simulink model "doc_design_iteration_viterbi_rayleigh_OFDM_MIMO"  (R2014a)
settings: Solver=FixedStepDiscrete  SolverMode=SingleTasking  StartTime=0.0  StopTime=inf  RelTol=1e-3
PostLoadFcn:
  | if ~exist('EbNo'),EbNo=6;end
  | if ~exist('maxNumBits'),maxNumBits=1e7;end;
  | if ~exist('maxNumErrs'),maxNumErrs=1e3;end;
  | 
  | load Parameters.mat
values from neighbouring files (symbols this model uses):
  EbNo = getTestParameter(obj,'EbNo')    [GrayCodedMod_EbNo_M.m]    (also in GrayCodedModulation2.m; commdoc_code.m = 10; commdoc_gray.m = 10; commdoc_mcurves.m = EbNoVec(idxEbNo))
  Peven = [1.41421356237 0 -1.41421356237 0 1.41421356237 0 -1.41421356237 0 1.41421356237 0 1.41421356237 0 ... (201 elements, 201x1)]    [Parameters.mat]
  Podd = [0 1.41421356237 0 1.41421356237 0 1.41421356237 0 1.41421356237 0 1.41421356237 0 -1.41421356237 ... (201 elements, 201x1)]    [Parameters.mat]
undefined symbols (not defined in the file or in its folder): doppler, prm80216ds
libraries: dspmtrx3 x4, dspindex x3, commchan3 x2, commdigbbndpm3 x2, commofdm x2, commcnvcod2 x2, commmimo x2, dspsigops x2, dspstat3 x1, dspmathops x1, commsink2 x1, commrandsrc2 x1
settings Model: Creator=The MathWorks Inc.
settings OptimizationCC: ExpressionDepthLimit=2147483647
settings DebuggingCC: UnderspecifiedInitializationDetection=Classic  SolverPrmCheckMsg=none  StateNameClashWarn=warning

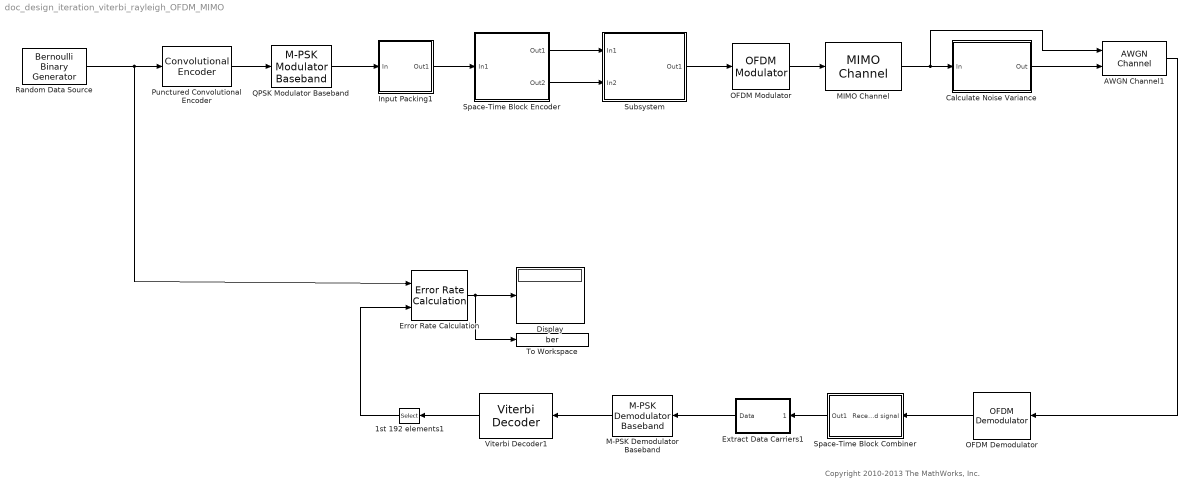
== system doc_design_iteration_viterbi_rayleigh_OFDM_MIMO ==
  note: Copyright 2010-2013 The MathWorks, Inc.
  1st 192 elements1 : Selector  NumberOfDimensions=2  InputPortWidth=3  IndexOptions=Index vector (dialog),Index vector (dialog)  Indices=1:378,1  OutputSizes=1,1
  AWGN Channel1 : commchan3/AWGN Channel  InputProcessing=Columns as channels (frame based)  seed=67  noiseMode=Variance from port  EbNodB=10  EsNodB=15  SNRdB=10  bitsPerSym=1  Ps=1  Tsym=1e-6  variance=1
  Calculate Noise Variance : Subsystem
      mask Display: disp('Calculate\nNoise Variance')
  Display : Display
  Error Rate Calculation : commsink2/Error Rate Calculation  N=0  st_delay=0  cp_mode=Entire frame  subframe=[]  PMode=Port  WsName=ErrorVec1  RsMode2=off  stop=on  numErr=maxNumErrs  maxBits=maxNumBits
  Extract Data Carriers1 : Subsystem  mask(OFDM Receiver){}
      mask Display: disp('Extract\nData Carriers');
  Input Packing1 : Subsystem
      mask Display: disp('IFFT Input\nPacking');
  M-PSK Demodulator Baseband : commdigbbndpm3/M-PSK Demodulator Baseband  M=4  Ph=pi/4  Dec=Gray  Mapping=[0 2 3 1]  OutType=Bit  DecType=Hard decision  VarSource=Dialog  Variance=1  outDtype1=boolean  outDtype2=Inherit via internal rule  derotateFactorWordLen=16
  MIMO Channel : commchan3/MIMO Channel  SimulateUsing=Code generation  SampleRate=3e6/25  PathDelays=[0 0.4 0.9]*1e-6  AveragePathGains=[0 -5 -10]  NormalizePathGains=on  FadingDistribution=Rayleigh  KFactor=3  DirectPathDopplerShift=0  DirectPathInitialPhase=0  MaximumDopplerShift=5  DopplerSpectrum=doppler( 'Jakes' )  SpatialCorrelation=on  NumTransmitAntennas=2  NumReceiveAntennas=1  TransmitCorrelationMatrix=[1 0; 0 1]  ReceiveCorrelationMatrix=1  AntennaSelection=Off  NormalizeChannelOutputs=on  RandomStream=mt19937ar with seed  Seed=73  PathGainsOutputPort=off
  OFDM Demodulator : commofdm/OFDM Demodulator  SimulateUsing=Code generation  FFTLength=256  NumGuardBandCarriers=[28; 27]  RemoveDCCarrier=off  PilotOutputPort=off  PilotCarrierIndices=[12; 26; 40; 54]  CyclicPrefixLength=32  NumSymbols=3  NumReceiveAntennas=1
  OFDM Modulator : commofdm/OFDM Modulator  SimulateUsing=Code generation  FFTLength=256  NumGuardBandCarriers=[28; 27]  InsertDCNull=off  PilotInputPort=off  PilotCarrierIndices=[12; 26; 40; 54]  CyclicPrefixLength=32  Windowing=off  WindowLength=1  NumSymbols=3  NumTransmitAntennas=2
  Punctured Convolutional Encoder : commcnvcod2/Convolutional Encoder  trellis=poly2trellis(7, [171 133])  opMode=Terminate trellis by appending bits  DelayedResetAction=off  hasIniStPort=off  hasFinStPort=off  usePuncVector=on  punctureVector=reshape([1 0;1 1],4,1)  reset=Unused parameter value
  QPSK Modulator Baseband : commdigbbndpm3/M-PSK Modulator Baseband  M=4  InType=Bit  Enc=Gray  Mapping=[0 2 3 1]  Ph=pi/4  outDtype=double  outWordLen=16  outUDDataType=sfix(16)  outFracLenMode=Best precision  outFracLen=15
  Random Data Source : commrandsrc2/Bernoulli Binary Generator  P=0.5  seed=61  Ts=25/3e6  frameBased=on  sampPerFrame=378  orient=off  outDataType=boolean
  Space-Time Block Encoder : Subsystem
      mask Display: disp('Space-Time\nDiversity\nEncoder');
  Space-Time Block Combiner : Subsystem
      mask Display: disp('Space-Time\nDiversity\nCombiner');
  Subsystem : Subsystem
      mask Display: disp('Add OFDM\nPreamble');
  To Workspace : ToWorkspace  VariableName=ber  SampleTime=-1
      settings: MaxDataPoints=1
  Viterbi Decoder1 : commcnvcod2/Viterbi Decoder  trellis=poly2trellis(7, [171 133])  isPunctured=off  punctureVector=reshape([1 0;1 1],4,1)  erasures=off  dectype=Hard decision  runSigValErrCheck=off  nsdecb=4  smWordLength=16  tbdepth=34  opmode=Terminated  reset=off  outDataType=boolean  delayedResetAction=off
  wires:
  Random Data Source/1 -> Error Rate Calculation/1, Punctured Convolutional Encoder/1
  Punctured Convolutional Encoder/1 -> QPSK Modulator Baseband/1
  QPSK Modulator Baseband/1 -> Input Packing1/1(In)
  Extract Data Carriers1/1(Data) -> M-PSK Demodulator Baseband/1
  M-PSK Demodulator Baseband/1 -> Viterbi Decoder1/1
  Viterbi Decoder1/1 -> 1st 192 elements1/1
  Input Packing1/1(Out1) -> Space-Time Block Encoder/1(In1)
  Space-Time Block Combiner/1(Out1) -> Extract Data Carriers1/1(Received signal)
  Error Rate Calculation/1 -> Display/1, To Workspace/1
  1st 192 elements1/1 -> Error Rate Calculation/2
  OFDM Modulator/1 -> MIMO Channel/1
  Subsystem/1(Out1) -> OFDM Modulator/1
  Space-Time Block Encoder/1(Out1) -> Subsystem/1(In1)
  Space-Time Block Encoder/2(Out2) -> Subsystem/2(In2)
  OFDM Demodulator/1 -> Space-Time Block Combiner/1(Received signal)
  MIMO Channel/1 -> Calculate Noise Variance/1(In), AWGN Channel1/1
  Calculate Noise Variance/1(Out) -> AWGN Channel1/2
  AWGN Channel1/1 -> OFDM Demodulator/1

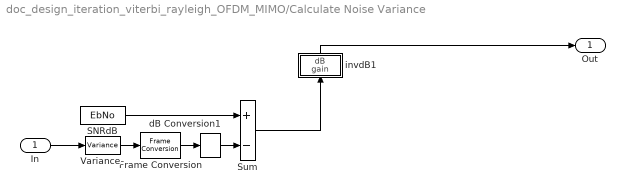
== system doc_design_iteration_viterbi_rayleigh_OFDM_MIMO/Calculate Noise Variance ==
  In : Inport
  Frame Conversion : FrameConversion  OutFrame=Sample-based
  SNRdB : Constant  Value=EbNo
  Sum : Sum  Inputs=+-  SaturateOnIntegerOverflow=on
  Variance : dspstat3/Variance  run=off  reset_popup=None  InputProcessing=Columns as channels (frame based)  directionMode=Each column  dimension=1  treatSBRowAsCol=on  roiEnable=off  roiType=Rectangles  roiPortion=Entire ROI  roiOutput=Individual statistics for each ROI  roiFlag=off  roundingMode=Floor  overflowMode=off
  dB Conversion1 : dspmathops/dB Conversion  dBtype=dB  intype=Power  R=1  fuzz=on
  invdB1 : Subsystem
      mask Display: disp('1/invdB')
  Out : Outport
  wires:
  dB Conversion1/1 -> Sum/2
  Variance/1 -> Frame Conversion/1
  Frame Conversion/1 -> dB Conversion1/1
  invdB1/1(dB) -> Out/1
  Sum/1 -> invdB1/1(gain)
  SNRdB/1 -> Sum/1
  In/1 -> Variance/1

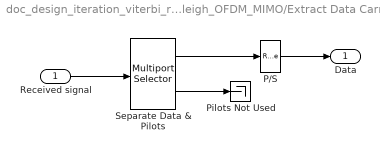
== system doc_design_iteration_viterbi_rayleigh_OFDM_MIMO/Extract Data Carriers1 ==
  Received signal : Inport
  P/S : Reshape  OutputDimensionality=Column vector (2-D)  OutputDimensions=[72, 1]
  Pilots Not Used : Terminator
  Separate Data & Pilots : dspindex/Multiport Selector  rowsOrCols=Rows  idxCellArray={[1:12 14:37 39:62 64:87 89:112 114:137 139:162 164:187 189:200],[13 38 63 88 113 138 163 188]}  idxErrMode=Clip Index
  Data : Outport
  wires:
  Received signal/1 -> Separate Data & Pilots/1
  Separate Data & Pilots/2 -> Pilots Not Used/1
  Separate Data & Pilots/1 -> P/S/1
  P/S/1 -> Data/1

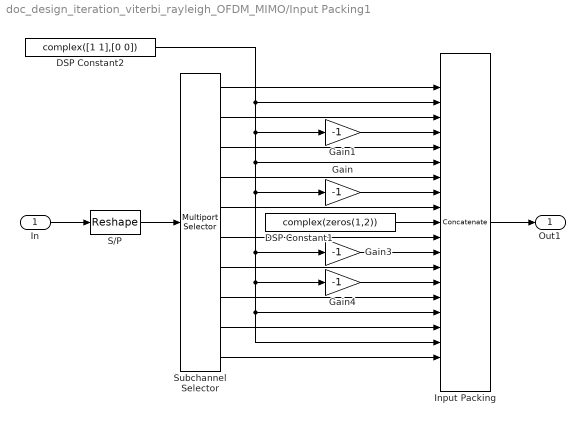
== system doc_design_iteration_viterbi_rayleigh_OFDM_MIMO/Input Packing1 ==
  In : Inport
  DSP Constant1 : Constant  Value=complex(zeros(1,2))  VectorParams1D=off
      settings: SamplingMode=Frame based
  DSP Constant2 : Constant  Value=complex([1 1],[0 0])  VectorParams1D=off
      settings: SamplingMode=Frame based
  Gain{,1,3..4} (4 alike) : Gain  Gain=-1
  Input Packing : Concatenate  NumInputs=19  Mode=Multidimensional array
  S/P : Reshape  OutputDimensionality=Customize  OutputDimensions=[192 2]
  Subchannel Selector : dspindex/Multiport Selector  rowsOrCols=Rows  idxCellArray={[1:12],[13:36],[37:60],[61:84],[85:96],[97:108],[109:132],[133:156],[157:180],[181:192]}  idxErrMode=Generate Error
  Out1 : Outport
  wires:
  Input Packing/1 -> Out1/1
  Gain4/1 -> Input Packing/14
  Gain3/1 -> Input Packing/12
  S/P/1 -> Subchannel Selector/1
  Gain1/1 -> Input Packing/4
  Gain/1 -> Input Packing/8
  DSP Constant1/1 -> Input Packing/10
  Subchannel Selector/1 -> Input Packing/1
  Subchannel Selector/2 -> Input Packing/3
  Subchannel Selector/3 -> Input Packing/5
  Subchannel Selector/4 -> Input Packing/7
  Subchannel Selector/5 -> Input Packing/9
  Subchannel Selector/6 -> Input Packing/11
  Subchannel Selector/7 -> Input Packing/13
  Subchannel Selector/8 -> Input Packing/15
  Subchannel Selector/9 -> Input Packing/17
  Subchannel Selector/10 -> Input Packing/19
  DSP Constant2/1 -> Input Packing/2, Input Packing/6, Gain3/1, Gain4/1, Input Packing/18, Input Packing/16, Gain/1, Gain1/1
  In/1 -> S/P/1

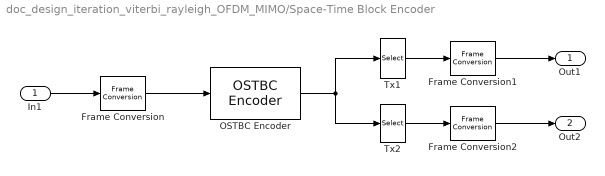
== system doc_design_iteration_viterbi_rayleigh_OFDM_MIMO/Space-Time Block Encoder ==
  In1 : Inport
  Frame Conversion : FrameConversion  OutFrame=Sample-based
  Frame Conversion1 : FrameConversion
  Frame Conversion2 : FrameConversion
  OSTBC Encoder : commmimo/OSTBC Encoder  numTx=2  rate=3/4  overflowMode=Wrap
  Tx1 : Selector  NumberOfDimensions=3  InputPortWidth=256  IndexOptions=Select all,Select all,Index vector (dialog)  Indices=prm80216ds.txCPIndices,1,1  OutputSizes=1,1,1
  Tx2 : Selector  NumberOfDimensions=3  InputPortWidth=256  IndexOptions=Select all,Select all,Index vector (dialog)  Indices=prm80216ds.txCPIndices,1,2  OutputSizes=1,1,1
  Out1 : Outport
  Out2 : Outport  Port=2
  wires:
  In1/1 -> Frame Conversion/1
  Frame Conversion1/1 -> Out1/1
  Frame Conversion2/1 -> Out2/1
  Tx1/1 -> Frame Conversion1/1
  Tx2/1 -> Frame Conversion2/1
  OSTBC Encoder/1 -> Tx1/1, Tx2/1
  Frame Conversion/1 -> OSTBC Encoder/1

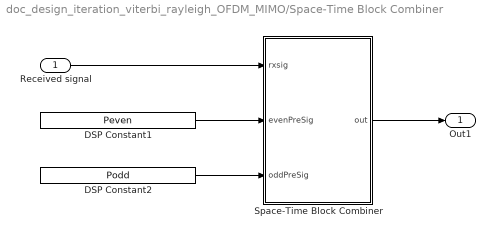
== system doc_design_iteration_viterbi_rayleigh_OFDM_MIMO/Space-Time Block Combiner ==
  Received signal : Inport
  DSP Constant1 : Constant  Value=Peven  VectorParams1D=off
      settings: SamplingMode=Frame based
  DSP Constant2 : Constant  Value=Podd  VectorParams1D=off
      settings: SamplingMode=Frame based
  Space-Time Block Combiner : Subsystem
      mask init:
      | a = [1:100; 1:100];
      mask Display: disp('Channel Estimation\n& Space-Time\nBlock Combining')
  Out1 : Outport
  wires:
  Space-Time Block Combiner/1(out) -> Out1/1
  Received signal/1 -> Space-Time Block Combiner/1(rxsig)
  DSP Constant2/1 -> Space-Time Block Combiner/3(oddPreSig)
  DSP Constant1/1 -> Space-Time Block Combiner/2(evenPreSig)

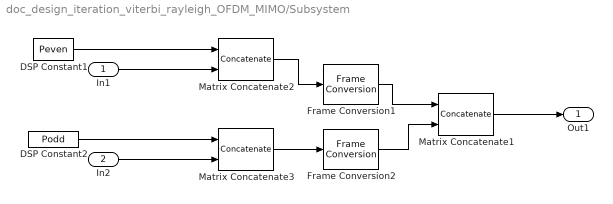
== system doc_design_iteration_viterbi_rayleigh_OFDM_MIMO/Subsystem ==
  In1 : Inport
  In2 : Inport  Port=2
  DSP Constant1 : Constant  Value=Peven  VectorParams1D=off
      settings: SamplingMode=Frame based
  DSP Constant2 : Constant  Value=Podd  VectorParams1D=off
      settings: SamplingMode=Frame based
  Frame Conversion1 : FrameConversion  OutFrame=Sample-based
  Frame Conversion2 : FrameConversion  OutFrame=Sample-based
  Matrix Concatenate1 : Concatenate  Mode=Multidimensional array  ConcatenateDimension=3
  Matrix Concatenate2 : Concatenate  Mode=Multidimensional array  ConcatenateDimension=2
  Matrix Concatenate3 : Concatenate  Mode=Multidimensional array  ConcatenateDimension=2
  Out1 : Outport
  wires:
  In2/1 -> Matrix Concatenate3/2
  In1/1 -> Matrix Concatenate2/2
  Matrix Concatenate1/1 -> Out1/1
  Frame Conversion1/1 -> Matrix Concatenate1/1
  Frame Conversion2/1 -> Matrix Concatenate1/2
  Matrix Concatenate3/1 -> Frame Conversion2/1
  Matrix Concatenate2/1 -> Frame Conversion1/1
  DSP Constant2/1 -> Matrix Concatenate3/1
  DSP Constant1/1 -> Matrix Concatenate2/1

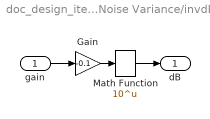
== system doc_design_iteration_viterbi_rayleigh_OFDM_MIMO/Calculate Noise Variance/invdB1 ==
  gain : Inport
  Gain : Gain  Gain=-0.1  SaturateOnIntegerOverflow=on  OutDataTypeStr=Inherit: Same as input  ParamDataTypeStr=Inherit: Same as input
  Math Function : Math  Operator=10^u  SaturateOnIntegerOverflow=on
  dB : Outport
  wires:
  Gain/1 -> Math Function/1
  gain/1 -> Gain/1
  Math Function/1 -> dB/1

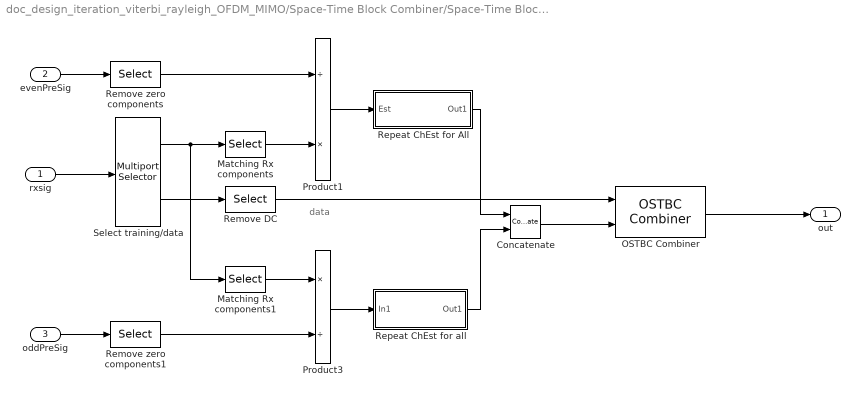
== system doc_design_iteration_viterbi_rayleigh_OFDM_MIMO/Space-Time Block Combiner/Space-Time Block Combiner ==
  note: data
  rxsig : Inport
  evenPreSig : Inport  Port=2
  oddPreSig : Inport  Port=3
  Concatenate : Concatenate  Mode=Multidimensional array  ConcatenateDimension=3
  Matching Rx components : Selector  NumberOfDimensions=2  InputPortWidth=53  IndexOptions=Index vector (dialog),Select all  Indices=[1:2:99 103:2:201],-1
  Matching Rx components1 : Selector  NumberOfDimensions=2  InputPortWidth=53  IndexOptions=Index vector (dialog),Select all  Indices=[2:2:201],-1
  OSTBC Combiner : commmimo/OSTBC Combiner  numTx=2  rate=3/4  numRx=1  roundingMode=Floor  overflowMode=Wrap  crossProductWordLen=32  crossProductFracLen=16  crossSumWordLen=32  crossSumFracLen=16  egyProductWordLen=32  egyProductFracLen=16  egySumWordLen=32  egySumFracLen=16  divisionWordLen=32  divisionFracLen=16
  Product1 : Product  Inputs=/*  SaturateOnIntegerOverflow=on  OutDataTypeStr=Inherit: Same as first input
  Product3 : Product  Inputs=*/  SaturateOnIntegerOverflow=on  OutDataTypeStr=Inherit: Same as first input
  "Remove DC " : Selector  NumberOfDimensions=2  InputPortWidth=53  IndexOptions=Index vector (dialog),Select all  Indices=[1:100 102:201],-1
  Remove zero components : Selector  NumberOfDimensions=2  InputPortWidth=53  IndexOptions=Index vector (dialog),Select all  Indices=[1:2:99 103:2:201],-1
  Remove zero components1 : Selector  NumberOfDimensions=2  InputPortWidth=53  IndexOptions=Index vector (dialog),Select all  Indices=[2:2:201],-1
  Repeat ChEst for All : Subsystem
  Repeat ChEst for all : Subsystem
  Select training/data : dspindex/Multiport Selector  rowsOrCols=Columns  idxCellArray={1,[2 3]}  idxErrMode=Clip Index
  out : Outport
  wires:
  Select training/data/2 -> "Remove DC "/1
  Product3/1 -> Repeat ChEst for all/1(In1)
  Matching Rx components1/1 -> Product3/1
  Remove zero components1/1 -> Product3/2
  oddPreSig/1 -> Remove zero components1/1
  Matching Rx components/1 -> Product1/2
  Remove zero components/1 -> Product1/1
  rxsig/1 -> Select training/data/1
  Product1/1 -> Repeat ChEst for All/1(Est)
  Select training/data/1 -> Matching Rx components1/1, Matching Rx components/1
  evenPreSig/1 -> Remove zero components/1
  OSTBC Combiner/1 -> out/1
  "Remove DC "/1 -> OSTBC Combiner/1
  Repeat ChEst for All/1(Out1) -> Concatenate/1
  Repeat ChEst for all/1(Out1) -> Concatenate/2
  Concatenate/1 -> OSTBC Combiner/2

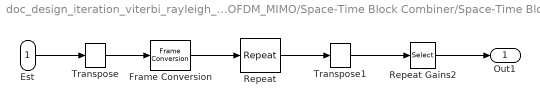
== system doc_design_iteration_viterbi_rayleigh_OFDM_MIMO/Space-Time Block Combiner/Space-Time Block Combiner/Repeat ChEst for All ==
  Est : Inport
  Frame Conversion : FrameConversion
  Repeat : dspsigops/Repeat  N=2  InputProcessing=Columns as channels (frame based)  RateOptions=Enforce single-rate processing  ic=0  mode=Unused parameter value
  Repeat Gains2 : Selector  NumberOfDimensions=2  InputPortWidth=53  IndexOptions=Index vector (dialog),Select all  Indices=a(:),-1
  Transpose : dspmtrx3/Transpose  Hermitian=off  overflowFlag=on
  Transpose1 : dspmtrx3/Transpose  Hermitian=off  overflowFlag=on
  Out1 : Outport
  wires:
  Frame Conversion/1 -> Repeat/1
  Repeat Gains2/1 -> Out1/1
  Est/1 -> Transpose/1
  Transpose1/1 -> Repeat Gains2/1
  Repeat/1 -> Transpose1/1
  Transpose/1 -> Frame Conversion/1

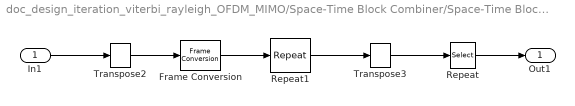
== system doc_design_iteration_viterbi_rayleigh_OFDM_MIMO/Space-Time Block Combiner/Space-Time Block Combiner/Repeat ChEst for all ==
  In1 : Inport
  Frame Conversion : FrameConversion
  Repeat : Selector  NumberOfDimensions=2  InputPortWidth=53  IndexOptions=Index vector (dialog),Select all  Indices=a(:),-1
  Repeat1 : dspsigops/Repeat  N=2  InputProcessing=Columns as channels (frame based)  RateOptions=Enforce single-rate processing  ic=0  mode=Unused parameter value
  Transpose2 : dspmtrx3/Transpose  Hermitian=off  overflowFlag=on
  Transpose3 : dspmtrx3/Transpose  Hermitian=off  overflowFlag=on
  Out1 : Outport
  wires:
  Frame Conversion/1 -> Repeat1/1
  Repeat/1 -> Out1/1
  In1/1 -> Transpose2/1
  Transpose3/1 -> Repeat/1
  Repeat1/1 -> Transpose3/1
  Transpose2/1 -> Frame Conversion/1
